simulink model "IEEE9_BUS_with2VSC_VI_Working"  (R2019b)
settings: Solver=ode23tb  StartTime=0.0  StopTime=Tend  RelTol=1e-3
values from neighbouring files (symbols this model uses):
  C_4 = 0.1670*C_b    (= 1.00487241952e-06)    [Basic_Model_Works.m]    (also in VSC_GridFroming_Thesis_Script.m; VSC_GridFroming_Thesis_Script_withSynchMach.m)
  C_6 = 0.2835*C_b    (= 1.70587623314e-06)    [Basic_Model_Works.m]    (also in VSC_GridFroming_Thesis_Script.m; VSC_GridFroming_Thesis_Script_withSynchMach.m)
  C_8 = 0.2275*C_b    (= 1.36891302659e-06)    [Basic_Model_Works.m]    (also in VSC_GridFroming_Thesis_Script.m; VSC_GridFroming_Thesis_Script_withSynchMach.m)
  C_dc = 0.008*(n)    (= 1.6)    [Basic_Model_Works.m]    (also in VSC_GridFroming_Thesis_Script.m; VSC_GridFroming_Thesis_Script_withSynchMach.m)
  C_f = C_f_pu*C1_b    (= 0.0318309886184)    [Basic_Model_Works.m]    (also in VSC_GridFroming_Thesis_Script.m; VSC_GridFroming_Thesis_Script_withSynchMach.m)
  droop_percentage = 1    [Basic_Model_Works.m]    (also in VSC_GridFroming_Thesis_Script.m; VSC_GridFroming_Thesis_Script_withSynchMach.m = 5)
  f_b = 50    [Basic_Model_Works.m]    (also in VSC_GridFroming_Thesis_Script.m; VSC_GridFroming_Thesis_Script_withSynchMach.m)
  I_b_LV = S_b/(sqrt(3)*V1_rms)    [Basic_Model_Works.m]    (also in VSC_GridFroming_Thesis_Script.m; VSC_GridFroming_Thesis_Script_withSynchMach.m)
  i_ll = -1.15*(S_b/Vdc_n)-i_loss_dc    [Basic_Model_Works.m]    (also in VSC_GridFroming_Thesis_Script.m; VSC_GridFroming_Thesis_Script_withSynchMach.m)
  I_threshold = I_thresh    (= 1)    [Basic_Model_Works.m]    (also in VSC_GridFroming_Thesis_Script.m)
  i_ul = 1.15*(S_b/Vdc_n)+i_loss_dc    [Basic_Model_Works.m]    (also in VSC_GridFroming_Thesis_Script.m; VSC_GridFroming_Thesis_Script_withSynchMach.m)
  isatpu = 1.4    [Basic_Model_Works.m]    (also in VSC_GridFroming_Thesis_Script.m; VSC_GridFroming_Thesis_Script_withSynchMach.m = 1.2)
  k_dc = eta_1/(Vdc_n*m_p)    [Basic_Model_Works.m]    (also in VSC_GridFroming_Thesis_Script.m; VSC_GridFroming_Thesis_Script_withSynchMach.m)
  K_p = (1/Vdc_n)    [Basic_Model_Works.m]    (also in VSC_GridFroming_Thesis_Script.m; VSC_GridFroming_Thesis_Script_withSynchMach.m)
  K_r = 1/R_dc    [Basic_Model_Works.m]    (also in VSC_GridFroming_Thesis_Script.m; VSC_GridFroming_Thesis_Script_withSynchMach.m)
  K_RV = 0.09    [Basic_Model_Works.m]    (also in VSC_GridFroming_Thesis_Script.m)
  Kff_i = 1    [Basic_Model_Works.m]    (also in VSC_GridFroming_Thesis_Script.m; VSC_GridFroming_Thesis_Script_withSynchMach.m)
  Kff_v = 1    [Basic_Model_Works.m]    (also in VSC_GridFroming_Thesis_Script.m; VSC_GridFroming_Thesis_Script_withSynchMach.m)
  Ki_i = (1/n)*1.19    (= 0.00595)    [Basic_Model_Works.m]    (also in VSC_GridFroming_Thesis_Script.m; VSC_GridFroming_Thesis_Script_withSynchMach.m)
  Ki_v = (n)*1.16    (= 232)    [Basic_Model_Works.m]    (also in VSC_GridFroming_Thesis_Script.m; VSC_GridFroming_Thesis_Script_withSynchMach.m = 232.2044)
  ki_v_ac = 10    [Basic_Model_Works.m]    (also in VSC_GridFroming_Thesis_Script.m; VSC_GridFroming_Thesis_Script_withSynchMach.m)
  Kp_i = 0.73    [Basic_Model_Works.m]    (also in VSC_GridFroming_Thesis_Script.m; VSC_GridFroming_Thesis_Script_withSynchMach.m = 0.738891)
  Kp_v = 0.52    [Basic_Model_Works.m]    (also in VSC_GridFroming_Thesis_Script.m; VSC_GridFroming_Thesis_Script_withSynchMach.m)
  kp_v_ac = 0.05    [Basic_Model_Works.m]    (also in VSC_GridFroming_Thesis_Script.m; VSC_GridFroming_Thesis_Script_withSynchMach.m)
  kp_VI = (-b+sqrt(b^2-4*a*c))/(2*a)    [Basic_Model_Works.m]    (also in VSC_GridFroming_Thesis_Script.m)
  L1_pu = 1*0.0186/m    (= 0.000186)    [Basic_Model_Works.m]    (also in VSC_GridFroming_Thesis_Script.m; VSC_GridFroming_Thesis_Script_withSynchMach.m)
  L2_mh = 0.08    [Basic_Model_Works.m]    (also in VSC_GridFroming_Thesis_Script.m; VSC_GridFroming_Thesis_Script_withSynchMach.m)
  L_45 = L_lines(2)    [Basic_Model_Works.m]    (also in VSC_GridFroming_Thesis_Script.m; VSC_GridFroming_Thesis_Script_withSynchMach.m)
  L_56 = L_lines(3)    [Basic_Model_Works.m]    (also in VSC_GridFroming_Thesis_Script.m; VSC_GridFroming_Thesis_Script_withSynchMach.m)
  L_67 = L_lines(5)    [Basic_Model_Works.m]    (also in VSC_GridFroming_Thesis_Script.m; VSC_GridFroming_Thesis_Script_withSynchMach.m)
  L_78 = L_lines(6)    [Basic_Model_Works.m]    (also in VSC_GridFroming_Thesis_Script.m; VSC_GridFroming_Thesis_Script_withSynchMach.m)
  L_89 = L_lines(8)    [Basic_Model_Works.m]    (also in VSC_GridFroming_Thesis_Script.m; VSC_GridFroming_Thesis_Script_withSynchMach.m)
  L_94 = L_lines(9)    [Basic_Model_Works.m]    (also in VSC_GridFroming_Thesis_Script.m; VSC_GridFroming_Thesis_Script_withSynchMach.m)
  L_f = L_f_pu*L1_b    (= 4.77464829276e-06)    [Basic_Model_Works.m]    (also in VSC_GridFroming_Thesis_Script.m; VSC_GridFroming_Thesis_Script_withSynchMach.m)
  L_v = L_v_pu*L1_b    (= 9.54929658551e-06)    [Basic_Model_Works.m]    (also in VSC_GridFroming_Thesis_Script.m; VSC_GridFroming_Thesis_Script_withSynchMach.m = 1.59154943092e-07)
  m_p = (50*(1.025)-  50*(0.975))/(n*VSC_Pn)    (= 1.25e-08)    [Basic_Model_Works.m]    (also in VSC_GridFroming_Thesis_Script.m; VSC_GridFroming_Thesis_Script_withSynchMach.m)
  n = 200    [Basic_Model_Works.m]    (also in VSC_GridFroming_Thesis_Script.m; VSC_GridFroming_Thesis_Script_withSynchMach.m)
  Pn = 210* 1e6    (= 210000000)    [Basic_Model_Works.m]    (also in VSC_GridFroming_Thesis_Script.m; VSC_GridFroming_Thesis_Script_withSynchMach.m)
  ps = 0.67*Ptot_Load/n_gen    (= 0.5025)    [Basic_Model_Works.m]    (also in VSC_GridFroming_Thesis_Script.m = 0.6; VSC_GridFroming_Thesis_Script_withSynchMach.m = 0.65)
  R1_pu = 1*0.00734/m    (= 7.34e-05)    [Basic_Model_Works.m]    (also in VSC_GridFroming_Thesis_Script.m; VSC_GridFroming_Thesis_Script_withSynchMach.m)
  R2_mh = 0.0027    [Basic_Model_Works.m]    (also in VSC_GridFroming_Thesis_Script.m; VSC_GridFroming_Thesis_Script_withSynchMach.m)
  R_45 = R_lines(2)    [Basic_Model_Works.m]    (also in VSC_GridFroming_Thesis_Script.m; VSC_GridFroming_Thesis_Script_withSynchMach.m)
  R_56 = R_lines(3)    [Basic_Model_Works.m]    (also in VSC_GridFroming_Thesis_Script.m; VSC_GridFroming_Thesis_Script_withSynchMach.m)
  R_67 = R_lines(5)    [Basic_Model_Works.m]    (also in VSC_GridFroming_Thesis_Script.m; VSC_GridFroming_Thesis_Script_withSynchMach.m)
  R_78 = R_lines(6)    [Basic_Model_Works.m]    (also in VSC_GridFroming_Thesis_Script.m; VSC_GridFroming_Thesis_Script_withSynchMach.m)
  R_89 = R_lines(8)    [Basic_Model_Works.m]    (also in VSC_GridFroming_Thesis_Script.m; VSC_GridFroming_Thesis_Script_withSynchMach.m)
  R_94 = R_lines(9)    [Basic_Model_Works.m]    (also in VSC_GridFroming_Thesis_Script.m; VSC_GridFroming_Thesis_Script_withSynchMach.m)
  R_dc = (Vdc_n/(0.05*(S_b)/Vdc_n))    [Basic_Model_Works.m]    (also in VSC_GridFroming_Thesis_Script.m; VSC_GridFroming_Thesis_Script_withSynchMach.m)
  R_f = R_f_pu*Z1_b    (= 5e-05)    [Basic_Model_Works.m]    (also in VSC_GridFroming_Thesis_Script.m; VSC_GridFroming_Thesis_Script_withSynchMach.m)
  R_v = R_v_pu*Z1_b    (= 0.002)    [Basic_Model_Works.m]    (also in VSC_GridFroming_Thesis_Script.m; VSC_GridFroming_Thesis_Script_withSynchMach.m = 1e-05)
  S_b = 100*(10^6)    (= 100000000)    [Basic_Model_Works.m]    (also in VSC_GridFroming_Thesis_Script.m; VSC_GridFroming_Thesis_Script_withSynchMach.m)
  T1sc_off = 13.15    [Basic_Model_Works.m]    (also in VSC_GridFroming_Thesis_Script.m)
  T1sc_on = 13    [Basic_Model_Works.m]    (also in VSC_GridFroming_Thesis_Script.m)
  T3sc_off = 30.15    [Basic_Model_Works.m]    (also in VSC_GridFroming_Thesis_Script.m)
  T3sc_on = 30    [Basic_Model_Works.m]    (also in VSC_GridFroming_Thesis_Script.m)
  T_en = T_conn-0.5    (= 12.5)    [Basic_Model_Works.m]    (also in VSC_GridFroming_Thesis_Script.m; VSC_GridFroming_Thesis_Script_withSynchMach.m = 11.5)
  T_s = 1e-4    (= 0.0001)    [Basic_Model_Works.m]    (also in VSC_GridFroming_Thesis_Script.m; VSC_GridFroming_Thesis_Script_withSynchMach.m)
  tau_dc = 0.05    [Basic_Model_Works.m]    (also in VSC_GridFroming_Thesis_Script.m; VSC_GridFroming_Thesis_Script_withSynchMach.m)
  tau_g = 0.25    [Basic_Model_Works.m]    (also in VSC_GridFroming_Thesis_Script.m; VSC_GridFroming_Thesis_Script_withSynchMach.m = 5)
  Tsc_off = 21.15    [Basic_Model_Works.m]    (also in VSC_GridFroming_Thesis_Script.m; VSC_GridFroming_Thesis_Script_withSynchMach.m = 20.25)
  Tsc_on = 21    [Basic_Model_Works.m]    (also in VSC_GridFroming_Thesis_Script.m; VSC_GridFroming_Thesis_Script_withSynchMach.m = 20)
  V = 230*(10^3)    (= 230000)    [Basic_Model_Works.m]    (also in VSC_GridFroming_Thesis_Script.m; VSC_GridFroming_Thesis_Script_withSynchMach.m)
  V1_rms = 1000    [Basic_Model_Works.m]    (also in VSC_GridFroming_Thesis_Script.m; VSC_GridFroming_Thesis_Script_withSynchMach.m)
  V2_rms = 13800    [Basic_Model_Works.m]    (also in VSC_GridFroming_Thesis_Script.m; VSC_GridFroming_Thesis_Script_withSynchMach.m)
  V_m = sqrt(2/3)*V1_rms    [Basic_Model_Works.m]    (also in VSC_GridFroming_Thesis_Script.m; VSC_GridFroming_Thesis_Script_withSynchMach.m)
  Vdc_n = 3*V_m    [Basic_Model_Works.m]    (also in VSC_GridFroming_Thesis_Script.m; VSC_GridFroming_Thesis_Script_withSynchMach.m)
  w_c = w_ref/4.95    (= 63.4665182543)    [Basic_Model_Works.m]    (also in VSC_GridFroming_Thesis_Script.m; VSC_GridFroming_Thesis_Script_withSynchMach.m)
  w_f = 7.5    [Basic_Model_Works.m]    (also in VSC_GridFroming_Thesis_Script.m; VSC_GridFroming_Thesis_Script_withSynchMach.m)
  w_ref = 2*pi*f_b    (= 314.159265359)    [Basic_Model_Works.m]    (also in VSC_GridFroming_Thesis_Script.m; VSC_GridFroming_Thesis_Script_withSynchMach.m)
  W_RV = 16.66    [Basic_Model_Works.m]    (also in VSC_GridFroming_Thesis_Script.m)
  XR = 3    [Basic_Model_Works.m]    (also in VSC_GridFroming_Thesis_Script.m; VSC_GridFroming_Thesis_Script_withSynchMach.m = 5)
undefined symbols (not defined in the file or in its folder): D1, Delta, i_dc
libraries: powerlib x78, powerlib_meascontrol x20, cstblocks x3, simulink x2, sps_avr x1
(part 1 of 3)
settings Model: SimulationMode=accelerator  ExtModeTrigDuration=100  Creator=TayyebiA  LastModifiedBy=carimjimenez
settings SolverCC: MaxConsecutiveMinStep=100
settings DataIOCC: SaveOutput=off  ReturnWorkspaceOutputs=off  StateSaveName=tmp_raccel_xout  SignalLoggingName=tmp_raccel_logsout
settings OptimizationCC: EfficientMapNaN2IntZero=off
settings DebuggingCC: ArithmeticOperatorsInVariantConditions=warning
settings HardwareCC: TargetBitPerLong=64  TargetBitPerPointer=64  TargetBitPerSizeT=64  TargetBitPerPtrDiffT=64  TargetLongLongMode=on  TargetIntDivRoundTo=Zero  TargetEndianess=LittleEndian  TargetWordSize=64  TargetHWDeviceType=MATLAB Host  ProdEqTarget=off
settings SFSimCC: SimUseLocalCustomCode=off  CustomCodeUndefinedFunction=UseInterfaceOnly
settings RTWCC: SystemTargetFile=accel.tlc  TemplateMakefile=accel_default_tmf  RTWVerbose=off  RTWUseLocalCustomCode=off
settings CodeAppCC: MaxIdLength=128
settings STFCustomTargetCC: ConcurrentExecutionCompliant=on  MATLABClassNameForMDSCustomization=Simulink.SoftwareTarget.TargetSpecificTriggerConfigurationBase  GRTInterface=on  SystemTargetFile=accel.tlc

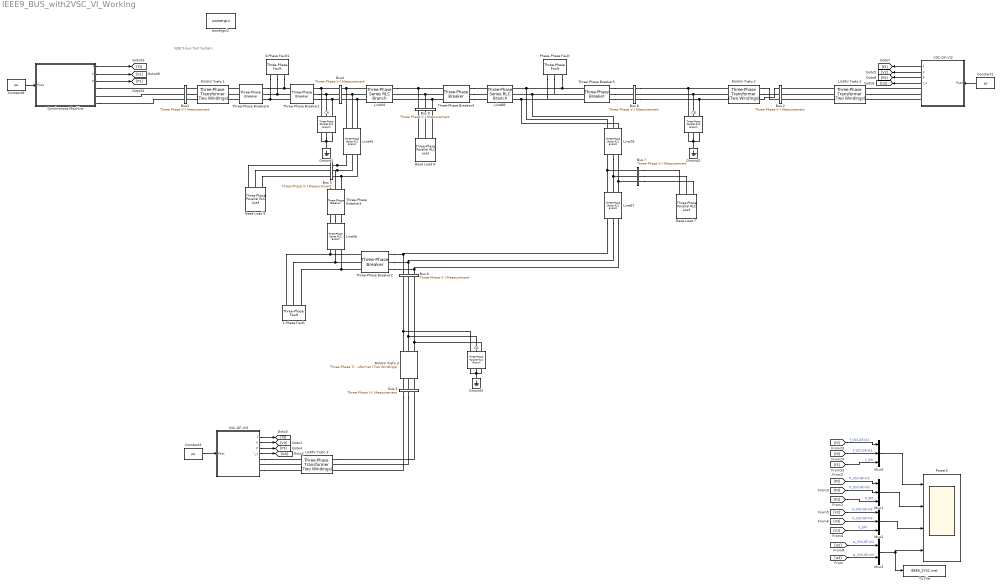
== system IEEE9_BUS_with2VSC_VI_Working ==
  note: IEEE 9-bus Test System
  1-Phase Fault : powerlib/Elements/Three-Phase Fault  InitialStates=0  FaultA=on  FaultB=off  FaultC=off  GroundFault=on  SwitchTimes=[T1sc_on T1sc_off]  External=off  SwitchStatus=NaN  FaultResistance=0.001  GroundResistance=1  SnubberResistance=1e6  SnubberCapacitance=inf  Measurements=None
      settings: SourceProductName=Simscape Electrical
  3-Phase Fault1 : powerlib/Elements/Three-Phase Fault  InitialStates=0  FaultA=on  FaultB=on  FaultC=on  GroundFault=on  SwitchTimes="[T3sc_on  T3sc_off]"  External=off  SwitchStatus=NaN  FaultResistance=0.001  GroundResistance=1  SnubberResistance=1e6  SnubberCapacitance=inf  Measurements=None
      settings: SourceProductName=Simscape Electrical
  Base Load 5 : powerlib/Elements/Three-Phase Parallel RLC Load  LConnTagsString=A|B|C  Configuration=Y (grounded)  NominalVoltage=V  Vabc=[1e3 1e3 1e3]  Vabcp=[1e3 1e3 1e3]  NominalFrequency=f_b  UnbalancedPower=off  ActivePower=pl  InductivePower=ql  CapacitivePower=0  Pabc=[10e3 9e3 11e3]  QLabc=[100 90 110]  QCabc=[100 90 110]  Pabcp=[10e3 9e3 11e3]  QLabcp=[100 90 110]  QCabcp=[100 90 110]  Measurements=None  LoadType=constant Z
      settings: SourceProductName=Simscape Electrical
  Base Load 7 : powerlib/Elements/Three-Phase Parallel RLC Load  LConnTagsString=A|B|C  Configuration=Y (grounded)  NominalVoltage=V  Vabc=[1e3 1e3 1e3]  Vabcp=[1e3 1e3 1e3]  NominalFrequency=f_b  UnbalancedPower=off  ActivePower=pl  InductivePower=ql  CapacitivePower=0  Pabc=[10e3 9e3 11e3]  QLabc=[100 90 110]  QCabc=[100 90 110]  Pabcp=[10e3 9e3 11e3]  QLabcp=[100 90 110]  QCabcp=[100 90 110]  Measurements=None  LoadType=constant Z
      settings: SourceProductName=Simscape Electrical
  "Base Load 9 " : powerlib/Elements/Three-Phase Parallel RLC Load  LConnTagsString=A|B|C  Configuration=Y (grounded)  NominalVoltage=V  Vabc=[1e3 1e3 1e3]  Vabcp=[1e3 1e3 1e3]  NominalFrequency=f_b  UnbalancedPower=off  ActivePower=pl  InductivePower=ql  CapacitivePower=0  Pabc=[10e3 9e3 11e3]  QLabc=[100 90 110]  QCabc=[100 90 110]  Pabcp=[10e3 9e3 11e3]  QLabcp=[100 90 110]  QCabcp=[100 90 110]  Measurements=None  LoadType=constant Z
      settings: SourceProductName=Simscape Electrical
  Bus 2 : powerlib/Measurements/Three-Phase V-I Measurement  VoltageMeasurement=no  SetLabelV=on  LabelV=Vabc_8  Vpu=on  VpuLL=off  CurrentMeasurement=no  SetLabelI=on  LabelI=Iabc_8  Ipu=on  Pbase=S_b  Vbase=V_b  OutputType=Complex  PhasorSimulation=off  PSBequivalent=0
      settings: SourceProductName=Simscape Electrical
  Bus 3 : powerlib/Measurements/Three-Phase V-I Measurement  VoltageMeasurement=no  SetLabelV=off  LabelV=Vabc_6  Vpu=off  VpuLL=off  CurrentMeasurement=no  SetLabelI=off  LabelI=Iabc_6  Ipu=off  Pbase=S_b  Vbase=V_b  OutputType=Complex  PhasorSimulation=off  PSBequivalent=0
      settings: SourceProductName=Simscape Electrical
  Bus 5 : powerlib/Measurements/Three-Phase V-I Measurement  VoltageMeasurement=no  SetLabelV=on  LabelV=Vabc_5  Vpu=on  VpuLL=off  CurrentMeasurement=no  SetLabelI=on  LabelI=Iabc_5  Ipu=on  Pbase=S_b  Vbase=V_b  OutputType=Complex  PhasorSimulation=off  PSBequivalent=0
      settings: SourceProductName=Simscape Electrical
  Bus 6 : powerlib/Measurements/Three-Phase V-I Measurement  VoltageMeasurement=no  SetLabelV=off  LabelV=Vabc_6  Vpu=off  VpuLL=off  CurrentMeasurement=no  SetLabelI=off  LabelI=Iabc_6  Ipu=off  Pbase=S_b  Vbase=V_b  OutputType=Complex  PhasorSimulation=off  PSBequivalent=0
      settings: SourceProductName=Simscape Electrical
  Bus 7 : powerlib/Measurements/Three-Phase V-I Measurement  VoltageMeasurement=no  SetLabelV=on  LabelV=Vabc_5  Vpu=on  VpuLL=off  CurrentMeasurement=no  SetLabelI=on  LabelI=Iabc_5  Ipu=on  Pbase=S_b  Vbase=V_b  OutputType=Complex  PhasorSimulation=off  PSBequivalent=0
      settings: SourceProductName=Simscape Electrical
  Bus 8 : powerlib/Measurements/Three-Phase V-I Measurement  VoltageMeasurement=no  SetLabelV=on  LabelV=Vabc_8  Vpu=on  VpuLL=off  CurrentMeasurement=no  SetLabelI=on  LabelI=Iabc_8  Ipu=on  Pbase=S_b  Vbase=V_b  OutputType=Complex  PhasorSimulation=off  PSBequivalent=0
      settings: SourceProductName=Simscape Electrical
  Bus 9 : powerlib/Measurements/Three-Phase V-I Measurement  VoltageMeasurement=no  SetLabelV=on  LabelV=Vabc_9  Vpu=on  VpuLL=off  CurrentMeasurement=no  SetLabelI=on  LabelI=Iabc_9  Ipu=on  Pbase=S_b  Vbase=V_b  OutputType=Complex  PhasorSimulation=off  PSBequivalent=0
      settings: SourceProductName=Simscape Electrical
  Bus1 : powerlib/Measurements/Three-Phase V-I Measurement  VoltageMeasurement=no  SetLabelV=on  LabelV=Vabc_1  Vpu=on  VpuLL=off  CurrentMeasurement=no  SetLabelI=on  LabelI=Iabc_1  Ipu=on  Pbase=S_b  Vbase=V_b  OutputType=Complex  PhasorSimulation=off  PSBequivalent=0
      settings: SourceProductName=Simscape Electrical
  Bus4 : powerlib/Measurements/Three-Phase V-I Measurement  VoltageMeasurement=no  SetLabelV=on  LabelV=Vabc_4  Vpu=on  VpuLL=off  CurrentMeasurement=no  SetLabelI=on  LabelI=Iabc_4  Ipu=on  Pbase=S_b  Vbase=V_b  OutputType=Complex  PhasorSimulation=off  PSBequivalent=0
      settings: SourceProductName=Simscape Electrical
  C4 : powerlib/Elements/Three-Phase Parallel RLC Branch  LConnTagsString=A|B|C  RConnTagsString=A|B|C  BranchType=C  Resistance=1  Inductance=1e-3  Capacitance=C_4  Measurements=None
      settings: SourceProductName=Simscape Electrical  SourceProductBaseCode=PS
  C6 : powerlib/Elements/Three-Phase Parallel RLC Branch  LConnTagsString=A|B|C  RConnTagsString=A|B|C  BranchType=C  Resistance=1  Inductance=1e-3  Capacitance=C_6  Measurements=None
      settings: SourceProductName=Simscape Electrical  SourceProductBaseCode=PS
  C8 : powerlib/Elements/Three-Phase Parallel RLC Branch  LConnTagsString=A|B|C  RConnTagsString=A|B|C  BranchType=C  Resistance=1  Inductance=1e-3  Capacitance=C_8  Measurements=None
      settings: SourceProductName=Simscape Electrical  SourceProductBaseCode=PS
  Constant1 : Constant  Value=ps
  Constant3 : Constant  Value=ps
  Constant8 : Constant  Value=ps
  Ground1 : powerlib/Elements/Ground  LConnTagsString=a
      settings: SourceProductName=Simscape Electrical
  Ground2 : powerlib/Elements/Ground  LConnTagsString=a
      settings: SourceProductName=Simscape Electrical
  Ground3 : powerlib/Elements/Ground  LConnTagsString=a
      settings: SourceProductName=Simscape Electrical
  LV/MV Trafo 2 : powerlib/Elements/Three-Phase Transformer (Two Windings)  Winding1Connection=Yg  Winding2Connection=Yg  CoreType=Three single-phase transformers  SetSaturation=off  Hysteresis=off  DataFile='hysteresis'  SetInitialFlux=off  Measurements=None  UNITS=pu  NominalPower=[S_b 50 ]  Winding1="[ V1_rms R1_pu  L1_pu]"  Winding2=[ V2_rms R1_pu L1_pu]  Rm=Rm_pu  Lm=Lm_pu  L0=0.5  Saturation="[ 0,0  ;  0.005,1.2  ;  1.0,1.4 ]"  InitialFluxes=[ 0.8 , -0.8 , 0.7 ]  BreakLoop=off  DiscreteSolver=Trapezoidal iterative  DataType=off  TransfoNumber=0
      settings: SourceProductName=Simscape Electrical
  LV/MV Trafo 3 : powerlib/Elements/Three-Phase Transformer (Two Windings)  Winding1Connection=Yg  Winding2Connection=Yg  CoreType=Three single-phase transformers  SetSaturation=off  Hysteresis=off  DataFile='hysteresis'  SetInitialFlux=off  Measurements=None  UNITS=pu  NominalPower=[S_b f_b ]  Winding1="[ V1_rms R1_pu  L1_pu]"  Winding2=[ V2_rms R1_pu L1_pu]  Rm=Rm_pu  Lm=Lm_pu  L0=0.5  Saturation="[ 0,0  ;  0.005,1.2  ;  1.0,1.4 ]"  InitialFluxes=[ 0.8 , -0.8 , 0.7 ]  BreakLoop=off  DiscreteSolver=Trapezoidal iterative  DataType=off  TransfoNumber=0
      settings: SourceProductName=Simscape Electrical
  Line45 : powerlib/Elements/Three-Phase Series RLC Branch  LConnTagsString=A|B|C  RConnTagsString=A|B|C  BranchType=RL  Resistance=R_45  Inductance=L_45  Capacitance=0  Measurements=None
      settings: SourceProductName=Simscape Electrical
  Line56 : powerlib/Elements/Three-Phase Series RLC Branch  LConnTagsString=A|B|C  RConnTagsString=A|B|C  BranchType=RL  Resistance=R_56  Inductance=L_56  Capacitance=0  Measurements=None
      settings: SourceProductName=Simscape Electrical
  Line67 : powerlib/Elements/Three-Phase Series RLC Branch  LConnTagsString=A|B|C  RConnTagsString=A|B|C  BranchType=RL  Resistance=R_67  Inductance=L_67  Capacitance=0  Measurements=None
      settings: SourceProductName=Simscape Electrical
  Line78 : powerlib/Elements/Three-Phase Series RLC Branch  LConnTagsString=A|B|C  RConnTagsString=A|B|C  BranchType=RL  Resistance=R_78  Inductance=L_78  Capacitance=0  Measurements=None
      settings: SourceProductName=Simscape Electrical
  Line89 : powerlib/Elements/Three-Phase Series RLC Branch  LConnTagsString=A|B|C  RConnTagsString=A|B|C  BranchType=RL  Resistance=R_89  Inductance=L_89  Capacitance=0  Measurements=None
      settings: SourceProductName=Simscape Electrical
  Line94 : powerlib/Elements/Three-Phase Series RLC Branch  LConnTagsString=A|B|C  RConnTagsString=A|B|C  BranchType=RL  Resistance=R_94  Inductance=L_94  Capacitance=0  Measurements=None
      settings: SourceProductName=Simscape Electrical
  "MV/HV Trafo 1 " : powerlib/Elements/Three-Phase Transformer (Two Windings)  Winding1Connection=Delta (D1)  Winding2Connection=Yg  CoreType=Three single-phase transformers  SetSaturation=off  Hysteresis=off  DataFile='hysteresis'  SetInitialFlux=off  Measurements=None  UNITS=pu  NominalPower=[ Pn f_b ]  Winding1=[V2_rms R2_mh L2_mh]  Winding2=[V R2_mh L2_mh]  Rm=Rm_mh  Lm=Lm_mh  L0=0.5  Saturation="[ 0,0  ;  0.005,1.2  ;  1.0,1.4 ]"  InitialFluxes=[ 0.8 , -0.8 , 0.7 ]  BreakLoop=off  DiscreteSolver=Trapezoidal iterative  DataType=off  TransfoNumber=0
      settings: SourceProductName=Simscape Electrical
  MV/HV Trafo 2 : powerlib/Elements/Three-Phase Transformer (Two Windings)  Winding1Connection=Delta (D1)  Winding2Connection=Yg  CoreType=Three single-phase transformers  SetSaturation=off  Hysteresis=off  DataFile='hysteresis'  SetInitialFlux=off  Measurements=None  UNITS=pu  NominalPower=[ Pn f_b ]  Winding1=[V2_rms R2_mh L2_mh]  Winding2=[V R2_mh L2_mh]  Rm=Rm_mh  Lm=Lm_mh  L0=0.5  Saturation="[ 0,0  ;  0.005,1.2  ;  1.0,1.4 ]"  InitialFluxes=[ 0.8 , -0.8 , 0.7 ]  BreakLoop=off  DiscreteSolver=Trapezoidal iterative  DataType=off  TransfoNumber=0
      settings: SourceProductName=Simscape Electrical
  "MV/HV Trafo 3 " : powerlib/Elements/Three-Phase Transformer (Two Windings)  Winding1Connection=Yg  Winding2Connection=Yg  CoreType=Three single-phase transformers  SetSaturation=off  Hysteresis=off  DataFile='hysteresis'  SetInitialFlux=off  Measurements=None  UNITS=pu  NominalPower=[ 210e6 50 ]  Winding1=[V2_rms 0.0027 0.08]  Winding2=[230e3 0.0027 0.08]  Rm=500  Lm=500  L0=0.5  Saturation="[ 0,0  ;  0.005,1.2  ;  1.0,1.4 ]"  InitialFluxes=[ 0.8 , -0.8 , 0.7 ]  BreakLoop=off  DiscreteSolver=Trapezoidal iterative  DataType=off  TransfoNumber=0
      settings: SourceProductName=Simscape Electrical
  Mux1 : Mux  Inputs=3
  Mux2 : Mux  Inputs=3
  Mux3 : Mux  Inputs=2
  Mux6 : Mux  Inputs=3
  Phase-Phase Fault : powerlib/Elements/Three-Phase Fault  InitialStates=0  FaultA=on  FaultB=on  FaultC=off  GroundFault=off  SwitchTimes=[Tsc_on Tsc_off]  External=off  SwitchStatus=NaN  FaultResistance=0.001  GroundResistance=1  SnubberResistance=1e6  SnubberCapacitance=inf  Measurements=None
      settings: SourceProductName=Simscape Electrical
  Power2 : Scope  NumInputPorts=4
  Synchronous Machine : Subsystem
  Three-Phase Breaker{1..6} (6 alike) : powerlib/Elements/Three-Phase Breaker  InitialState=open  SwitchA=on  SwitchB=on  SwitchC=on  SwitchTimes=[0]  External=off  BreakerResistance=0.01  SnubberResistance=1e6  SnubberCapacitance=inf  Measurements=None
      settings: SourceProductName=Simscape Electrical
  To File : ToFile  Filename=IEEE9_2VSC.mat  MatrixName=Is_VSC
  VSC-GF-VI2 : Subsystem
  VSC-GF-VI3 : Subsystem
  powergui2 : powerlib/powergui  Priority=1  SimulationMode=Discrete  SampleTime=T_s  frequency=50  Iterations=50  frequencyindice=0  Pbase=100e6  ErrMax=0.0001  UnitsV=kV  UnitsW=MW  buscounter=0  FunctionMessages=off  echomessages=off  EnableUseOfTLC=off  CurrentSourceSwitches=off  DisableSnubberDevices=off  DisableRonSwitches=off  DisableVfSwitches=off  DisplayEquations=off  AutomaticDiscreteSolvers=off  SolverType=Tustin/Backward Euler (TBE)  Interpol=off  ExternalGateDelay=off  methode=off  Ts=100  x0status=blocks  SPID=off  SwTol=0  HookPort=off  NonlinearTolerance=1e-4  nMaxIteration=100  ContinueOnMaxIteration=off  RestoreLinks=warning  ResistiveCurrentMeasurement=off  Frange=[0:2:500]  Ylog=off  Xlog=on  ShowGrid=off  save=off  variable=ZData  structure=0  ZoomFFT=off  StartTime=0.0  cycles=1  DisplayStyle=1  fundamental=60  FreqAxis=off  MaxFrequency=1000  frequencyindicesteady=1  RmsSteady=1  display=off
      settings: SourceProductName=Simscape Electrical
  wires:
  [P3] -> Mux1/2  "P_VSC-GF-VI3"
  [V3] -> Mux2/2  "V_VSC-GF-VI3"
  Mux6/1 -> Power2/1
  Mux1/1 -> Power2/2
  Mux2/1 -> Power2/3
  Mux3/1 -> To File/1, Power2/4
  [Is3] -> Mux3/2  "Is_VSC-GF-VI3"
  Constant8/1 -> Synchronous Machine/1(Pset)
  [Is2] -> Mux3/1  "Is_VSC-GF-VI2"
  Constant3/1 -> VSC-GF-VI3/1(Pset)
  Constant1/1 -> VSC-GF-VI2/1(Pset)
  [f2] -> Mux6/1  "f_VSC-GF-VI2"
  [f3] -> Mux6/2  "f_VSC-GF-VI3"
  [P2] -> Mux1/1  "P_VSC-GF-VI2"
  [V2] -> Mux2/1  "V_VSC-GF-VI2"
  VSC-GF-VI2/1(f) -> [f2]
  VSC-GF-VI2/2(V) -> [V2]
  VSC-GF-VI2/3(P) -> [P2]
  VSC-GF-VI2/4(I_s) -> [Is2]
  VSC-GF-VI3/3(P) -> [P3]
  VSC-GF-VI3/4(I_s) -> [Is3]
  VSC-GF-VI3/2(V) -> [V3]
  VSC-GF-VI3/1(f) -> [f3]
  Synchronous Machine/1(f) -> [f1]
  Synchronous Machine/2(V) -> [V1]
  Synchronous Machine/3(P) -> [P1]
  [f1] -> Mux6/3  "f_SM"
  [P1] -> Mux1/3  "P_SM"
  [V1] -> Mux2/3  "V_SM"
  connections:
  "MV/HV Trafo 3 "/RConn2 -- C6/LConn2 -- Bus 6/RConn2
  Bus 7/LConn2 -- Base Load 7/LConn2
  Line78/LConn2 -- Three-Phase Breaker5/LConn2 -- Phase-Phase Fault/LConn2 -- Line89/RConn2
  Bus 8/LConn3 -- MV/HV Trafo 2/RConn3 -- C8/LConn3
  Bus 9/RConn2 -- Three-Phase Breaker4/LConn2 -- Line94/RConn2
  Bus 7/LConn3 -- Base Load 7/LConn3
  Line67/LConn1 -- Bus 7/RConn1 -- Line78/RConn1
  Bus 5/LConn3 -- Three-Phase Breaker3/RConn3 -- Line45/RConn3
  Line94/RConn1 -- Three-Phase Breaker4/LConn1 -- Bus 9/RConn3
  C4/RConn2 -- C4/RConn3 -- Ground1/LConn1 -- C4/RConn1
  Bus 8/LConn1 -- MV/HV Trafo 2/RConn1 -- C8/LConn1
  C8/LConn2 -- MV/HV Trafo 2/RConn2 -- Bus 8/LConn2
  C8/RConn3 -- Ground2/LConn1 -- C8/RConn2 -- C8/RConn1
  Line67/RConn2 -- Three-Phase Breaker2/RConn2 -- Bus 6/LConn2
  C4/LConn1 -- Three-Phase Breaker1/RConn1 -- Bus4/RConn1
  Bus4/LConn1 -- Line45/LConn1 -- Line94/LConn1
  C6/LConn3 -- "MV/HV Trafo 3 "/RConn3 -- Bus 6/RConn3
  "MV/HV Trafo 3 "/RConn1 -- C6/LConn1 -- Bus 6/RConn1
  Bus4/LConn2 -- Line45/LConn2 -- Line94/LConn2
  Line78/LConn3 -- Three-Phase Breaker5/LConn3 -- Phase-Phase Fault/LConn3 -- Line89/RConn3
  Phase-Phase Fault/LConn1 -- Three-Phase Breaker5/LConn1 -- Line89/RConn1 -- Line78/LConn1
  Bus4/RConn3 -- Three-Phase Breaker1/RConn3 -- C4/LConn3
  Bus 5/LConn1 -- Three-Phase Breaker3/RConn1 -- Line45/RConn1
  Bus 9/RConn1 -- Three-Phase Breaker4/LConn3 -- Line94/RConn3
  Line67/RConn3 -- Three-Phase Breaker2/RConn3 -- Bus 6/LConn3
  Bus4/LConn3 -- Line45/LConn3 -- Line94/LConn3
  Bus4/RConn2 -- Three-Phase Breaker1/RConn2 -- C4/LConn2
  Bus 5/LConn2 -- Three-Phase Breaker3/RConn2 -- Line45/RConn2
  "Base Load 9 "/LConn1 -- Bus 9/LConn3
  "Base Load 9 "/LConn3 -- Bus 9/LConn1
  "Base Load 9 "/LConn2 -- Bus 9/LConn2
  "MV/HV Trafo 1 "/LConn1 -- Bus1/LConn1
  "MV/HV Trafo 1 "/LConn2 -- Bus1/LConn2
  "MV/HV Trafo 1 "/LConn3 -- Bus1/LConn3
  Bus 3/RConn1 -- LV/MV Trafo 3/RConn1
  Bus 3/RConn2 -- LV/MV Trafo 3/RConn2
  LV/MV Trafo 3/RConn3 -- Bus 3/RConn3
  Bus 3/LConn1 -- "MV/HV Trafo 3 "/LConn1
  Bus 3/LConn2 -- "MV/HV Trafo 3 "/LConn2
  Bus 3/LConn3 -- "MV/HV Trafo 3 "/LConn3
  Bus 7/LConn1 -- Base Load 7/LConn1
  Line67/LConn3 -- Bus 7/RConn3 -- Line78/RConn3
  Line78/RConn2 -- Bus 7/RConn2 -- Line67/LConn2
  C6/RConn1 -- Ground3/LConn1 -- C6/RConn2 -- C6/RConn3
  3-Phase Fault1/LConn1 -- Three-Phase Breaker6/RConn1 -- Three-Phase Breaker1/LConn1
  3-Phase Fault1/LConn2 -- Three-Phase Breaker6/RConn2 -- Three-Phase Breaker1/LConn2
  3-Phase Fault1/LConn3 -- Three-Phase Breaker6/RConn3 -- Three-Phase Breaker1/LConn3
  LV/MV Trafo 2/RConn3 -- Bus 2/LConn1
  Bus 2/LConn2 -- LV/MV Trafo 2/RConn2
  LV/MV Trafo 2/RConn1 -- Bus 2/LConn3
  MV/HV Trafo 2/LConn2 -- Bus 2/RConn2
  MV/HV Trafo 2/LConn1 -- Bus 2/RConn3
  Bus 2/RConn1 -- MV/HV Trafo 2/LConn3
  Bus 5/RConn3 -- Base Load 5/LConn3
  Bus 5/RConn2 -- Base Load 5/LConn2
  Bus 5/RConn1 -- Base Load 5/LConn1
  VSC-GF-VI2/RConn1 -- LV/MV Trafo 2/LConn3
  LV/MV Trafo 2/LConn2 -- VSC-GF-VI2/RConn2
  VSC-GF-VI2/RConn3 -- LV/MV Trafo 2/LConn1
  VSC-GF-VI3/RConn1 -- LV/MV Trafo 3/LConn3
  LV/MV Trafo 3/LConn2 -- VSC-GF-VI3/RConn2
  VSC-GF-VI3/RConn3 -- LV/MV Trafo 3/LConn1
  Synchronous Machine/RConn1 -- Bus1/RConn1
  Bus1/RConn2 -- Synchronous Machine/RConn2
  Synchronous Machine/RConn3 -- Bus1/RConn3
  Line67/RConn1 -- Three-Phase Breaker2/RConn1 -- Bus 6/LConn1
  Three-Phase Breaker3/LConn1 -- Line56/LConn1
  Three-Phase Breaker3/LConn2 -- Line56/LConn2
  Line56/LConn3 -- Three-Phase Breaker3/LConn3
  Three-Phase Breaker5/RConn2 -- Bus 8/RConn2
  Three-Phase Breaker5/RConn1 -- Bus 8/RConn1
  Three-Phase Breaker5/RConn3 -- Bus 8/RConn3
  Three-Phase Breaker4/RConn1 -- Line89/LConn1
  Three-Phase Breaker4/RConn2 -- Line89/LConn2
  Three-Phase Breaker4/RConn3 -- Line89/LConn3
  Three-Phase Breaker6/LConn1 -- "MV/HV Trafo 1 "/RConn1
  Three-Phase Breaker6/LConn2 -- "MV/HV Trafo 1 "/RConn2
  Three-Phase Breaker6/LConn3 -- "MV/HV Trafo 1 "/RConn3
  1-Phase Fault/LConn3 -- Three-Phase Breaker2/LConn3 -- Line56/RConn3
  Three-Phase Breaker2/LConn2 -- 1-Phase Fault/LConn2 -- Line56/RConn2
  1-Phase Fault/LConn1 -- Line56/RConn1 -- Three-Phase Breaker2/LConn1

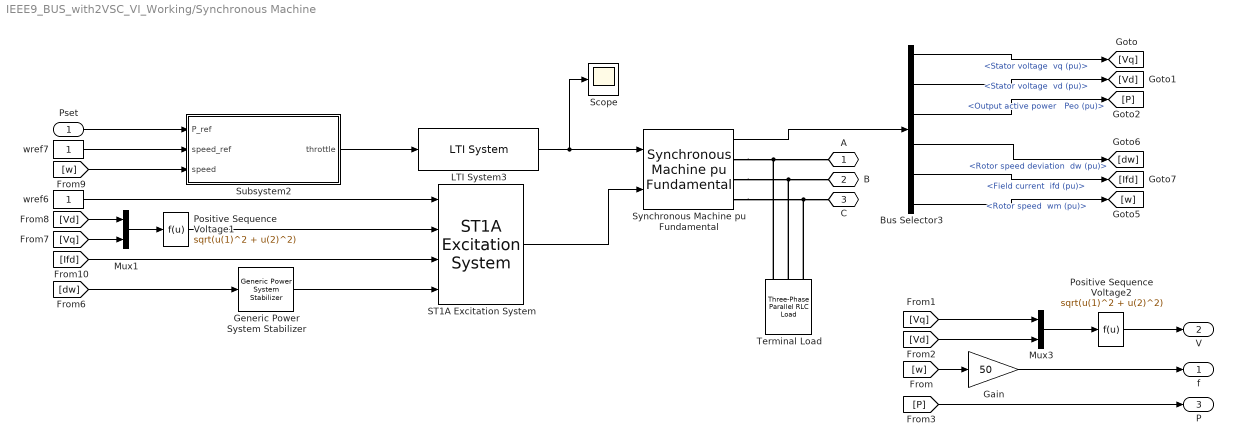
== system IEEE9_BUS_with2VSC_VI_Working/Synchronous Machine ==
  Pset : Inport
  Bus Selector3 : BusSelector  OutputSignals="dq0 components.Stator voltage  vq (pu),dq0 components.Stator voltage  vd (pu),Output active power   Peo (pu),Mechanical.Rotor speed deviation  dw (pu),dq0 components.Field current  ifd (pu),Mechanical.Rotor speed  wm (pu)"
  Gain : Gain  Gain=50
  Generic Power System Stabilizer : powerlib/Machines/Generic Power System Stabilizer  Tsensor=30e-4  K=2.5  Twashout=2  Tleadlag1=[2*50e-3 0.1*20e-3]  Tleadlag2=[2*3 0.1*5.4]  VSlimits=2*[-0.15 0.15]  Vinit=0  Plot_On=off  MagdB_On=on  FreqRange=logspace(-2,2,500)
      settings: SourceProductName=Simscape Electrical  SourceProductBaseCode=PS
  LTI System3 : cstblocks/LTI System  sys=ss(-1/tau_g,1/tau_g,1,[])  IC=ps
  Mux1 : Mux  Inputs=2
  Mux3 : Mux  Inputs=2
  Positive Sequence Voltage1 : Fcn  Expr=sqrt(u(1)^2 + u(2)^2)
  Positive Sequence Voltage2 : Fcn  Expr=sqrt(u(1)^2 + u(2)^2)
  ST1A Excitation System : sps_avr/ST1A Excitation System  Tr=20e-3  KaTa=[210 0.001]  VIminmax=[-999 +999]  VAminmax=[-999 999]  VRminmax=[-6.0 6.43]  KfTf=[0.001 1]  TbTc=[0 0 0 0]  KLR=1  ILR=2  Kc=0.038  v0=[1 1]  TsBlock=0
      settings: SourceProductName=Simscape Electrical  SourceProductBaseCode=PS
  Scope : Scope
  Subsystem2 : Subsystem
  Synchronous Machine pu Fundamental : powerlib/Machines/Synchronous Machine pu Fundamental  PresetModel=No  MechanicalLoad=Mechanical power Pm  ShowDetailedParameters=on  RotorType=Salient-pole  Units=per unit fundamental parameters  MeasurementBus=off  NominalParameters="[100E6  V2_rms   50]"  Stator="[ 2.85E-03  0.114  1.19  0.36 ]"  Field="[ 5.79E-04  0.114]"  Dampers2=[0.0652, 0.5134, 0.0287, 0.2553, 7.765e-3, 0.9167 ]  Dampers1="[ 1.17E-02  0.182  1.97E-02  0.384 ]"  Mechanical=[ 3.7 0 20]  PolePairs=20  InitialConditions="[ 0  0  0  0  0  0  0  0  1 ]"  SetSaturation=off  Saturation=[0.6404,0.7127,0.8441,0.9214,0.9956,1.082,1.19,1.316,1.457;0.7,0.7698,0.8872,0.9466,0.9969,1.046,1.1,1.151,1.201]  LoadFlowParameters=[1,0,0,0,0]  TsPowergui=0  TsBlock=-1  IterativeModel=Trapezoidal non iterative  IterativeDiscreteModel=Trapezoidal non iterative  BusType=PV  Pref=0  Qref=0  Qmin=-inf  Qmax=inf  PLF=0  QLF=0
      settings: SourceProductName=Simscape Electrical  SourceProductBaseCode=PS
  Terminal Load : powerlib/Elements/Three-Phase Parallel RLC Load  LConnTagsString=A|B|C  Configuration=Y (grounded)  NominalVoltage=V2_rms  Vabc=[1e3 1e3 1e3]  Vabcp=[1e3 1e3 1e3]  NominalFrequency=50  UnbalancedPower=off  ActivePower=1  InductivePower=0  CapacitivePower=0  Pabc=[10e3 9e3 11e3]  QLabc=[100 90 110]  QCabc=[100 90 110]  Pabcp=[10e3 9e3 11e3]  QLabcp=[100 90 110]  QCabcp=[100 90 110]  Measurements=None  LoadType=constant Z
      settings: SourceProductName=Simscape Electrical
  wref6 : Constant
  wref7 : Constant
  A : PMIOPort  Side=Right
  B : PMIOPort  Port=2  Side=Right
  C : PMIOPort  Port=3  Side=Right
  f : Outport  VectorParamsAs1DForOutWhenUnconnected=off
  V : Outport  Port=2  VectorParamsAs1DForOutWhenUnconnected=off
  P : Outport  Port=3  VectorParamsAs1DForOutWhenUnconnected=off
  wires:
  Gain/1 -> f/1
  Pset/1 -> Subsystem2/1(P_ref)
  Positive Sequence Voltage2/1 -> V/1
  wref7/1 -> Subsystem2/2(speed_ref)
  wref6/1 -> ST1A Excitation System/1
  Mux3/1 -> Positive Sequence Voltage2/1
  Synchronous Machine pu Fundamental/1 -> Bus Selector3/1
  [w] -> Gain/1
  [Vq] -> Mux3/1
  [Vd] -> Mux3/2
  [P] -> P/1
  [w] -> Subsystem2/3(speed)
  Subsystem2/1(throttle) -> LTI System3/1
  Bus Selector3/1 -> [Vq]  "<Stator voltage  vq (pu)>"
  Bus Selector3/2 -> [Vd]  "<Stator voltage  vd (pu)>"
  Bus Selector3/3 -> [P]  "<Output active power   Peo (pu)>"
  Bus Selector3/4 -> [dw]  "<Rotor speed deviation  dw (pu)>"
  Bus Selector3/5 -> [Ifd]  "<Field current  ifd (pu)>"
  Bus Selector3/6 -> [w]  "<Rotor speed  wm (pu)>"
  LTI System3/1 -> Scope/1, Synchronous Machine pu Fundamental/1
  Generic Power System Stabilizer/1 -> ST1A Excitation System/4
  [dw] -> Generic Power System Stabilizer/1
  [Ifd] -> ST1A Excitation System/3
  Mux1/1 -> Positive Sequence Voltage1/1
  [Vd] -> Mux1/1
  [Vq] -> Mux1/2
  Positive Sequence Voltage1/1 -> ST1A Excitation System/2
  ST1A Excitation System/1 -> Synchronous Machine pu Fundamental/2
  connections:
  Terminal Load/LConn1 -- Synchronous Machine pu Fundamental/RConn1 -- A/RConn1
  Terminal Load/LConn3 -- Synchronous Machine pu Fundamental/RConn3 -- C/RConn1
  Terminal Load/LConn2 -- Synchronous Machine pu Fundamental/RConn2 -- B/RConn1

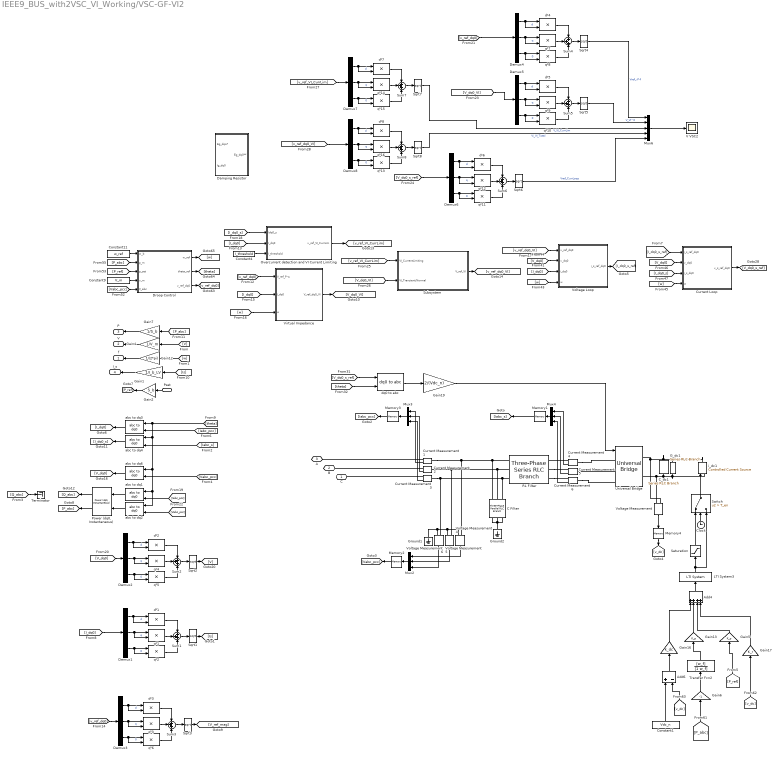
== system IEEE9_BUS_with2VSC_VI_Working/VSC-GF-VI2 ==
  Pset : Inport
  " Virtual Impedance" : Subsystem
  Add4 : Sum  Inputs=++++
  Add6 : Sum  Inputs=+-
  C Filter : powerlib/Elements/Three-Phase Parallel RLC Branch  LConnTagsString=A|B|C  RConnTagsString=A|B|C  BranchType=C  Resistance=1  Inductance=1e-3  Capacitance=C_f  Measurements=None
      settings: SourceProductName=Simscape Electrical  SourceProductBaseCode=PS
  C_dc1 : powerlib/Elements/Series RLC Branch  LConnTagsString=__new0  RConnTagsString=__new0  BranchType=C  Resistance=1  Inductance=1e-3  SetiL0=off  InitialCurrent=0  Capacitance=C_dc  Setx0=off  InitialVoltage=Vdc_n  Measurements=None
      settings: SourceProductName=Simscape Electrical
  Clock : Clock
  Constant1 : Constant  Value=Vdc_n
  Constant11 : Constant  Value=w_ref
  Constant4 : Constant  Value=I_threshold
  Constant9 : Constant  Value=V_m
  Current Loop : Subsystem
  Current Measurement{1..6} (6 alike) : powerlib/Measurements/Current Measurement  PhasorSimulation=off  OutputType=Complex  PSBequivalent=0
      settings: SourceProductName=Simscape Electrical
  Damping Resistor : Subsystem
  Demux{1..8} (8 alike) : Demux  Outputs=3
  Droop Control : Subsystem
  G_dc1 : powerlib/Elements/Series RLC Branch  LConnTagsString=__new0  RConnTagsString=__new0  BranchType=R  Resistance=R_dc  Inductance=1e-3  SetiL0=off  InitialCurrent=0  Capacitance=1e-6  Setx0=off  InitialVoltage=0  Measurements=None
      settings: SourceProductName=Simscape Electrical
  Gain1 : Gain  Gain=1/I_b_LV
  Gain12 : Gain  Gain=1/(2*pi)
  Gain13 : Gain  Gain=K_p
  Gain16 : Gain  Gain=k_dc
  Gain17 : Gain  Gain=K_r
  Gain19 : Gain  Gain=2/(Vdc_n)
  Gain2 : Gain  Gain=S_b
  Gain4 : Gain  Gain=1/V_m
  Gain5 : Gain  Gain=K_p
  Gain6 : Gain  Gain=-1
  Gain7 : Gain  Gain=1/S_b
  Ground1 : powerlib/Elements/Ground  LConnTagsString=a
      settings: SourceProductName=Simscape Electrical
  Ground2 : powerlib/Elements/Ground  LConnTagsString=a
      settings: SourceProductName=Simscape Electrical
  LTI System3 : cstblocks/LTI System  sys=tf(1,[tau_dc 1])  IC=[]
  Memory{1..4} (4 alike) : Memory
  Mux2 : Mux  Inputs=3
  Mux3 : Mux  Inputs=3
  Mux4 : Mux  Inputs=3
  Mux6 : Mux  Inputs=5
  Overcurrent detection and VI Current Limiting : Subsystem
  "Power (dq0, Instantaneous)" : powerlib_meascontrol/Measurements/Power (dq0, Instantaneous)
      settings: SourceProductName=Simscape Electrical  SourceProductBaseCode=PS
  RL Filter : powerlib/Elements/Three-Phase Series RLC Branch  LConnTagsString=A|B|C  RConnTagsString=A|B|C  BranchType=RL  Resistance=R_f  Inductance=L_f  Capacitance=0  Measurements=None
      settings: SourceProductName=Simscape Electrical
  Saturation : Saturate  UpperLimit=i_ul  LowerLimit=i_ll
  Sqrt{1..8} (8 alike) : Sqrt  SaturateOnIntegerOverflow=on
  Subsystem : Subsystem
  Sum{1..8} (8 alike) : Sum  Inputs=+++  SaturateOnIntegerOverflow=on  InputSameDT=on  OutDataTypeStr=Inherit: Same as first input
  Switch : Switch  Criteria=u2 > Threshold  Threshold=T_en
  Terminator : Terminator
  Transfer Fcn2 : TransferFcn  Numerator=[w_f]  Denominator=[1 w_f]
  Universal Bridge : powerlib/Power Electronics/Universal Bridge  Arms=3  SnubberResistance=1e5  SnubberCapacitance=inf  Device=Average-model based VSC  Ron=1e-3  Lon=0  ForwardVoltages="[  0  0  ]"  ForwardVoltage=0  GTOparameters=[ 10e-6 , 20e-6 ]  IGBTparameters=[ 1e-6 , 2e-6 ]  Measurements=None  Measurements_2=None  converterType=Rectifier
      settings: SourceProductName=Simscape Electrical
  V VSC2 : Scope
  Voltage Loop : Subsystem
  Voltage Measurement{,4..6} (4 alike) : powerlib/Measurements/Voltage Measurement  PhasorSimulation=off  OutputType=Complex  PSBequivalent=0
      settings: SourceProductName=Simscape Electrical
  abc to dq{1..4,6} (5 alike) : powerlib_meascontrol/Transformations/abc to dq0  Alignment=90 degrees behind phase A axis
      settings: SourceProductName=Simscape Electrical
  dq0 to abc : powerlib_meascontrol/Transformations/dq0 to abc  Alignment=90 degrees behind phase A axis
      settings: SourceProductName=Simscape Electrical
  d²{1..8} (8 alike) : Product  SaturateOnIntegerOverflow=on  RndMeth=Zero  InputSameDT=on  OutDataTypeStr=Inherit: Same as first input
  i_dc1 : powerlib/Electrical Sources/Controlled Current Source  Initialize=off  Source_Type=DC  Amplitude=i_dc  Phase=0  Frequency=0  Measurements=None
      settings: SourceProductName=Simscape Electrical
  q²{1..16} (16 alike) : Product  SaturateOnIntegerOverflow=on  RndMeth=Zero  InputSameDT=on  OutDataTypeStr=Inherit: Same as first input
  C : PMIOPort  Side=Right
  B : PMIOPort  Port=2  Side=Right
  A : PMIOPort  Port=3  Side=Right
  f : Outport  VectorParamsAs1DForOutWhenUnconnected=off
  V : Outport  Port=2  VectorParamsAs1DForOutWhenUnconnected=off
  P : Outport  Port=3  VectorParamsAs1DForOutWhenUnconnected=off
  I_s : Outport  Port=4  VectorParamsAs1DForOutWhenUnconnected=off
  wires:
  Gain7/1 -> P/1
  [P_abc] -> Gain7/1
  Current Measurement6/1 -> Mux4/3
  Current Measurement5/1 -> Mux4/2
  Current Measurement4/1 -> Mux4/1
  Current Measurement3/1 -> Mux3/3
  Current Measurement2/1 -> Mux3/2
  Current Measurement1/1 -> Mux3/1
  Voltage Measurement4/1 -> Mux2/1
  Voltage Measurement5/1 -> Mux2/2
  Voltage Measurement6/1 -> Mux2/3
  [V] -> Gain4/1
  Gain2/1 -> [P_ref]
  Pset/1 -> Gain2/1
  Gain12/1 -> f/1
  [w] -> Gain12/1
  Mux2/1 -> Memory2/1
  Mux3/1 -> Memory3/1
  abc to dq1/1 -> "Power (dq0, Instantaneous)"/2
  abc to dq2/1 -> "Power (dq0, Instantaneous)"/1
  [Vabc_pcc] -> abc to dq2/1
  "Power (dq0, Instantaneous)"/2 -> [Q_abc]
  "Power (dq0, Instantaneous)"/1 -> [P_abc]
  [Iabc_pcc] -> abc to dq1/1
  Gain4/1 -> V/1
  [Iabc_pcc] -> abc to dq3/1
  [Iabc_s] -> abc to dq4/1
  [Vabc_pcc] -> abc to dq6/1
  [theta] -> abc to dq2/2, abc to dq1/2, abc to dq6/2, abc to dq4/2, abc to dq3/2
  abc to dq3/1 -> [I_dq0]
  abc to dq4/1 -> [I_dq0_s]
  abc to dq6/1 -> [V_dq0]
  [theta] -> dq0 to abc/2
  q²4/1 -> Sum2/2
  [V_dq0] -> Demux2/1
  q²5/1 -> Sum2/3
  Sum2/1 -> Sqrt2/1
  Demux2/3 -> q²5/1, q²5/2  "0"
  d²2/1 -> Sum2/1
  Demux2/2 -> q²4/1, q²4/2  "q"
  Demux2/1 -> d²2/1, d²2/2  "d"
  Sqrt2/1 -> [V]
  Mux4/1 -> Memory1/1
  Memory2/1 -> [Vabc_pcc]
  Memory3/1 -> [Iabc_pcc]
  Memory1/1 -> [Iabc_s]
  dq0 to abc/1 -> Gain19/1
  Switch/1 -> i_dc1/1
  Gain19/1 -> Universal Bridge/1
  [V_dq0_s_ref] -> dq0 to abc/1
  Gain16/1 -> Add4/1
  Gain6/1 -> Transfer Fcn2/1
  [P_ref] -> Gain5/1
  Memory4/1 -> [v_dc]
  Add4/1 -> LTI System3/1
  [v_dc] -> Gain17/1
  Gain13/1 -> Add4/2
  Add6/1 -> Gain16/1
  Voltage Measurement/1 -> Memory4/1
  Clock/1 -> Switch/2
  [P_abc] -> Gain6/1
  Constant1/1 -> Add6/1
  Gain5/1 -> Add4/3
  Gain17/1 -> Add4/4
  LTI System3/1 -> Switch/3, Saturation/1
  Transfer Fcn2/1 -> Gain13/1
  Saturation/1 -> Switch/1
  [v_dc] -> Add6/2
  [Q_abc] -> Terminator/1
  q²2/1 -> Sum1/3
  Demux1/2 -> q²1/1, q²1/2  "q"
  [I_dq0] -> Demux1/1
  Demux1/1 -> d²1/1, d²1/2  "d"
  Sum1/1 -> Sqrt1/1
  Demux1/3 -> q²2/1, q²2/2  "0"
  Sqrt1/1 -> [Is]
  d²1/1 -> Sum1/1
  q²1/1 -> Sum1/2
  [Is] -> Gain1/1
  Gain1/1 -> I_s/1
  [v_ref_dq0] -> Demux3/1
  Demux3/2 -> q²3/1, q²3/2  "q"
  Demux3/1 -> d²3/1, d²3/2  "d"
  q²3/1 -> Sum3/2
  q²6/1 -> Sum3/3
  Sum3/1 -> Sqrt3/1
  Demux3/3 -> q²6/1, q²6/2  "0"
  d²3/1 -> Sum3/1
  Sqrt3/1 -> [V_ref_mag]
  [P_abc] -> Droop Control/2(p_m)
  Constant9/1 -> Droop Control/4(v_m)
  Constant11/1 -> Droop Control/1(w_b)
  [Vabc_pcc] -> Droop Control/5(V_abc)
  Droop Control/2(theta_ref) -> [theta]
  Droop Control/1(w_ref) -> [w]
  [P_ref] -> Droop Control/3(p_set)
  Droop Control/3(v_ref_dq0) -> [v_ref_dq0]
  [v_ref_dq0_VI] -> Voltage Loop/1(v_ref_dq0)
  Demux4/1 -> d²4/1, d²4/2  "d"
  [V_dq0_VI] -> Subsystem/2(VI_Transient/Normal)
  q²13/1 -> Sum8/3
  [v_ref_dq0_VI] -> Demux8/1
  q²14/1 -> Sum7/2
  Demux6/3 -> q²11/1, q²11/2  "0"
  Constant4/1 -> Overcurrent detection and VI Current Limiting/3(I_threshold)
  Sqrt7/1 -> Mux6/3  "V_VI_CurrLim"
  Overcurrent detection and VI Current Limiting/1(v_ref_VI_CurrLim) -> [v_ref_VI_CurrLim]
  [V_dq0] -> Voltage Loop/2(v_dq0)
  Demux4/3 -> q²8/1, q²8/2  "0"
  q²12/1 -> Sum6/2
  q²8/1 -> Sum4/3
  Demux8/2 -> q²16/1, q²16/2  "q"
  Sqrt4/1 -> Mux6/1  "Vref_-P-f"
  [v_ref_dq0] -> Demux4/1
  [V_dq0_VI] -> Demux5/1
  [I_dq0_s] -> Current Loop/3(i_s_dq0)
  [I_dq0] -> " Virtual Impedance"/2(I_dq0)
  [w] -> Current Loop/4(w)
  Voltage Loop/1(i_s_ref_dq0) -> [I_dq0_s_ref]
  q²9/1 -> Sum5/2
  [v_ref_VI_CurrLim] -> Demux7/1
  Subsystem/1(V_ref_VI) -> [v_ref_dq0_VI]
  [I_dq0_s_ref] -> Current Loop/1(i_s_ref_dq0)
  Sum6/1 -> Sqrt6/1
  Sum8/1 -> Sqrt8/1
  [v_ref_VI_CurrLim] -> Subsystem/1(VI_CurrentLimiting)
  Sum4/1 -> Sqrt4/1
  Demux7/1 -> d²7/1, d²7/2  "d"
  [w] -> " Virtual Impedance"/3(w)
  Demux5/3 -> q²10/1, q²10/2  "0"
  Demux5/2 -> q²9/1, q²9/2  "q"
  Demux5/1 -> d²5/1, d²5/2  "d"
  d²7/1 -> Sum7/1
  [v_ref_dq0] -> " Virtual Impedance"/1("V_ref_P-w ")
  d²5/1 -> Sum5/1
  [I_dq0] -> Overcurrent detection and VI Current Limiting/2(I_dq0)
  q²10/1 -> Sum5/3
  Demux8/3 -> q²13/1, q²13/2  "0"
  Current Loop/1(v_s_ref_dq0) -> [V_dq0_s_ref]
  [w] -> Voltage Loop/4(w)
  [I_dq0_s] -> Overcurrent detection and VI Current Limiting/1(Idq0_s)
  Mux6/1 -> V VSC2/1
  d²6/1 -> Sum6/1
  d²4/1 -> Sum4/1
  Sqrt8/1 -> Mux6/4  "Vi_VI_Total"
  q²15/1 -> Sum7/3
  Demux6/1 -> d²6/1, d²6/2  "d"
  Demux7/2 -> q²14/1, q²14/2  "q"
  Demux7/3 -> q²15/1, q²15/2  "0"
  Demux6/2 -> q²12/1, q²12/2  "q"
  Sum7/1 -> Sqrt7/1
  Demux8/1 -> d²8/1, d²8/2  "d"
  d²8/1 -> Sum8/1
  q²16/1 -> Sum8/2
  Sqrt6/1 -> Mux6/5  "Vref_CurrLoop"
  [V_dq0] -> Current Loop/2(v_dq0)
  q²7/1 -> Sum4/2
  " Virtual Impedance"/1(V_ref_dq0_VI) -> [V_dq0_VI]
  q²11/1 -> Sum6/3
  Demux4/2 -> q²7/1, q²7/2  "q"
  [I_dq0] -> Voltage Loop/3(i_dq0)
  Sum5/1 -> Sqrt5/1
  [V_dq0_s_ref] -> Demux6/1
  Sqrt5/1 -> Mux6/2  "V_VI^0"
  connections:
  Current Measurement2/LConn1 -- C Filter/LConn2 -- RL Filter/RConn2 -- Voltage Measurement5/LConn1
  Voltage Measurement6/LConn1 -- RL Filter/RConn3 -- C Filter/LConn3 -- Current Measurement3/LConn1
  Universal Bridge/RConn1 -- i_dc1/RConn1 -- G_dc1/LConn1 -- C_dc1/LConn1 -- Voltage Measurement/LConn1
  Voltage Measurement6/LConn2 -- Voltage Measurement5/LConn2 -- Voltage Measurement4/LConn2 -- Ground1/LConn1
  Current Measurement3/RConn1 -- C/RConn1
  Current Measurement2/RConn1 -- B/RConn1
  Current Measurement1/RConn1 -- A/RConn1
  Current Measurement6/LConn1 -- Universal Bridge/LConn3
  Current Measurement5/LConn1 -- Universal Bridge/LConn2
  Current Measurement4/LConn1 -- Universal Bridge/LConn1
  Universal Bridge/RConn2 -- i_dc1/LConn1 -- G_dc1/RConn1 -- C_dc1/RConn1 -- Voltage Measurement/LConn2
  RL Filter/RConn1 -- C Filter/LConn1 -- Voltage Measurement4/LConn1 -- Current Measurement1/LConn1
  C Filter/RConn1 -- Ground2/LConn1 -- C Filter/RConn2 -- C Filter/RConn3
  Current Measurement4/RConn1 -- RL Filter/LConn1
  RL Filter/LConn2 -- Current Measurement5/RConn1
  RL Filter/LConn3 -- Current Measurement6/RConn1
